simulink model "Aufgabe_1_3"  (R2016b)
settings: Solver=VariableStepAuto  StartTime=0.0  StopTime=10.0  RelTol=1e-3
values from neighbouring files (symbols this model uses):
  x1_0 = 0    [aufgabe1.m]    (also in aufgabe3.m)
  x2_0 = 0    [aufgabe1.m]    (also in aufgabe3.m)
  x3_0 = 0    [aufgabe1.m]    (also in aufgabe3.m)
settings Model: Creator=M  LastModifiedBy=M

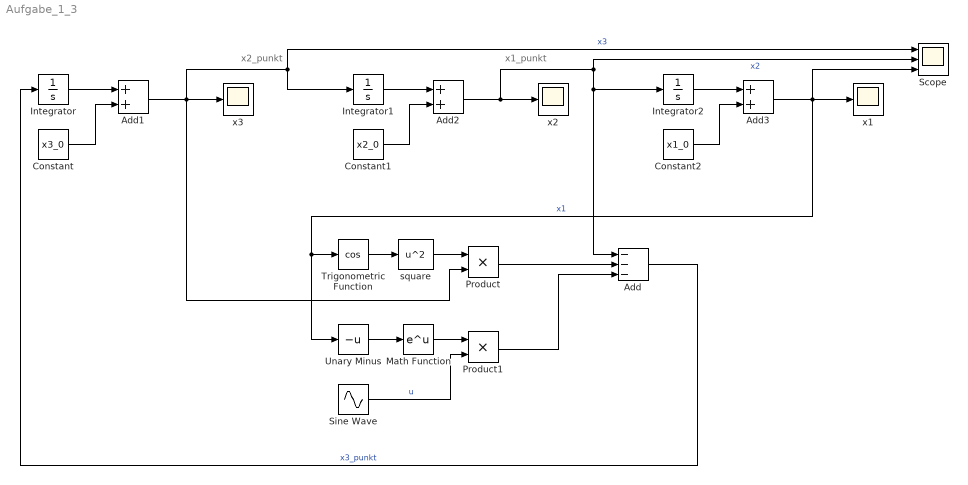
== system Aufgabe_1_3 ==
  note: x1_punkt
  note: x2_punkt
  Add : Sum  Inputs=---
  Add1 : Sum
  Add2 : Sum
  Add3 : Sum
  Constant : Constant  Value=x3_0
  Constant1 : Constant  Value=x2_0
  Constant2 : Constant  Value=x1_0
  Integrator : Integrator
  Integrator1 : Integrator
  Integrator2 : Integrator
  Math Function : Math  SaturateOnIntegerOverflow=on
  Product : Product
  Product1 : Product
  Scope : Scope  NumInputPorts=3
  Sine Wave : Sin  SampleTime=0
  Trigonometric Function : Trigonometry  Operator=cos
  Unary Minus : UnaryMinus
  square : Fcn  Expr=u^2
  x1 : Scope
  x2 : Scope
  x3 : Scope
  wires:
  Sine Wave/1 -> Product1/2  "u"
  Math Function/1 -> Product1/1
  Unary Minus/1 -> Math Function/1
  Integrator/1 -> Add1/1
  Constant/1 -> Add1/2
  Add1/1 -> x3/1, Integrator1/1, Scope/1, Product/2  "x3"
  Integrator1/1 -> Add2/1
  Constant1/1 -> Add2/2
  Add2/1 -> Add/1, Integrator2/1, Scope/2, x2/1  "x2"
  Integrator2/1 -> Add3/1
  Constant2/1 -> Add3/2
  Add3/1 -> Scope/3, Trigonometric Function/1, Unary Minus/1, x1/1  "x1"
  square/1 -> Product/1
  Product/1 -> Add/2
  Product1/1 -> Add/3
  Add/1 -> Integrator/1  "x3_punkt"
  Trigonometric Function/1 -> square/1
